simulink model "POWER_BTN_CONTROL"  (R2024b)
settings: configuration reference "MODEL_CONFIG_CHILD" (kept outside this file)
undefined symbols (not defined in the file): MILLI_SEC_COUNTS_10000_U16, MILLI_SEC_COUNTS_1000_U16, MILLI_SEC_COUNTS_2000_U16, SAMPLE_TIME_1MS
libraries: simulink x2
settings Model: DataDictionary=MCU_FOC_MAIN_DD.sldd  EnableAccessToBaseWorkspace=off  Creator=415  LastModifiedBy=415
settings ConfigSetRef: SourceName=MODEL_CONFIG_CHILD

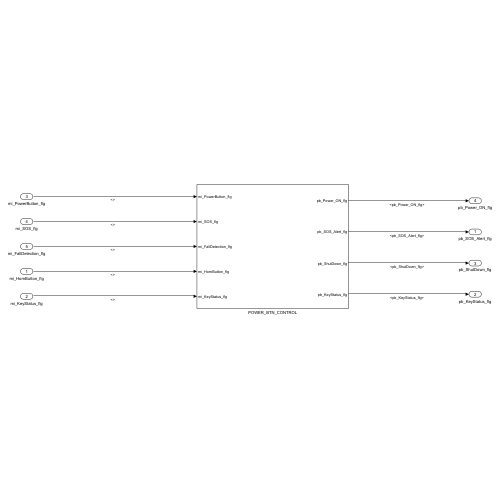
[thumbnail: Simulink's stored preview of the top-level diagram]
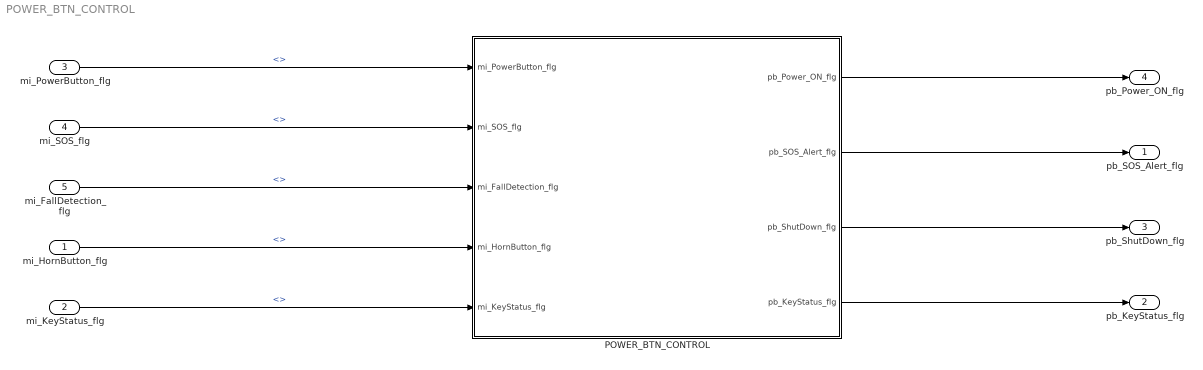
== system POWER_BTN_CONTROL ==
  mi_HornButton_flg : Inport
  mi_KeyStatus_flg : Inport  Port=2
  mi_PowerButton_flg : Inport  Port=3
  mi_SOS_flg : Inport  Port=4
  mi_FallDetection_flg : Inport  Port=5
  POWER_BTN_CONTROL : Subsystem
  pb_SOS_Alert_flg : Outport
  pb_KeyStatus_flg : Outport  Port=2
  pb_ShutDown_flg : Outport  Port=3
  pb_Power_ON_flg : Outport  Port=4
  wires:
  mi_PowerButton_flg/1 -> POWER_BTN_CONTROL/1(mi_PowerButton_flg)  "<>"
  POWER_BTN_CONTROL/3(pb_ShutDown_flg) -> pb_ShutDown_flg/1
  POWER_BTN_CONTROL/4(pb_KeyStatus_flg) -> pb_KeyStatus_flg/1
  POWER_BTN_CONTROL/1(pb_Power_ON_flg) -> pb_Power_ON_flg/1
  mi_KeyStatus_flg/1 -> POWER_BTN_CONTROL/5(mi_KeyStatus_flg)  "<>"
  POWER_BTN_CONTROL/2(pb_SOS_Alert_flg) -> pb_SOS_Alert_flg/1
  mi_FallDetection_flg/1 -> POWER_BTN_CONTROL/3(mi_FallDetection_flg)  "<>"
  mi_HornButton_flg/1 -> POWER_BTN_CONTROL/4(mi_HornButton_flg)  "<>"
  mi_SOS_flg/1 -> POWER_BTN_CONTROL/2(mi_SOS_flg)  "<>"

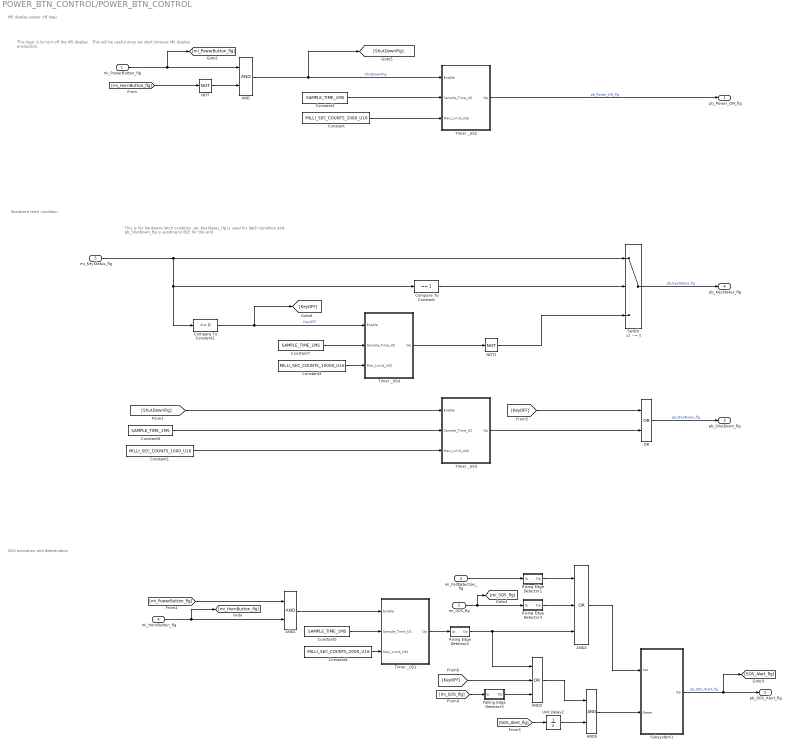
== system POWER_BTN_CONTROL/POWER_BTN_CONTROL ==
  note: This logic is to turn off the M5 display . This will be useful once we start inhouse M5 display production.
  note: M5 display power off logic
  note: This is for hardware latch condition .pb_KeyStatus_flg is used for latch condition and pb_ShutDown_flg is sending to BLE for trip end .
  note: Hardware latch condition
  note: SOS activation and deactivation
  mi_PowerButton_flg : Inport
  mi_SOS_flg : Inport  Port=2
  mi_FallDetection_flg : Inport  Port=3
  mi_HornButton_flg : Inport  Port=4
  mi_KeyStatus_flg : Inport  Port=5
  AND : Logic  AllPortsSameDT=off  OutDataTypeStr=boolean
  AND1 : Logic  AllPortsSameDT=off  OutDataTypeStr=boolean
  AND2 : Logic  Operator=OR  Inputs=3  AllPortsSameDT=off  OutDataTypeStr=boolean
  AND3 : Logic  Operator=OR  Inputs=3  AllPortsSameDT=off  OutDataTypeStr=boolean
  AND5 : Logic  AllPortsSameDT=off  OutDataTypeStr=boolean
  Compare To Constant : simulink/Logic and Bit Operations/Compare To Constant  relop===  const=1  OutDataTypeStr=boolean
  Compare To Constant1 : simulink/Logic and Bit Operations/Compare To Constant  relop===  const=0  OutDataTypeStr=boolean
  Constant : Constant  Value=MILLI_SEC_COUNTS_2000_U16
  Constant1 : Constant  Value=MILLI_SEC_COUNTS_1000_U16
  Constant{2,5,7..8} (4 alike) : Constant  Value=SAMPLE_TIME_1MS
  Constant3 : Constant  Value=MILLI_SEC_COUNTS_10000_U16
  Constant4 : Constant  Value=MILLI_SEC_COUNTS_2000_U16
  Falling Edge Detector3 : Subsystem
  NOT : Logic  Operator=NOT  AllPortsSameDT=off  OutDataTypeStr=boolean
  NOT1 : Logic  Operator=NOT  IconShape=distinctive  AllPortsSameDT=off  OutDataTypeStr=boolean
  OR : Logic  Operator=OR  AllPortsSameDT=off  OutDataTypeStr=boolean
  Rising Edge Detector1 : Subsystem
  Rising Edge Detector2 : Subsystem
  Rising Edge Detector3 : Subsystem
  Subsystem1 : Subsystem
  Switch : Switch  Criteria=u2 ~= 0  SaturateOnIntegerOverflow=off  InputSameDT=off
  Timer _US1 : Subsystem
  Timer _US2 : Subsystem
  Timer _US3 : Subsystem
  Timer _US4 : Subsystem
  Unit Delay2 : UnitDelay  SampleTime=-1  HasFrameUpgradeWarning=on
  pb_Power_ON_flg : Outport
  pb_SOS_Alert_flg : Outport  Port=2
  pb_ShutDown_flg : Outport  Port=3
  pb_KeyStatus_flg : Outport  Port=4
  wires:
  [KeyOFF] -> AND3/2
  OR/1 -> pb_ShutDown_flg/1  "pb_ShutDown_flg"
  [ShutDownFlg] -> Timer _US3/1(Enable)
  [KeyOFF] -> OR/1
  Compare To Constant/1 -> Switch/2
  Timer _US4/1(Op) -> NOT1/1
  NOT1/1 -> Switch/3
  Compare To Constant1/1 -> Timer _US4/1(Enable), [KeyOFF]  "KeyOFF"
  Switch/1 -> pb_KeyStatus_flg/1  "pb_KeyStatus_flg"
  mi_KeyStatus_flg/1 -> Compare To Constant/1, Compare To Constant1/1, Switch/1
  Constant7/1 -> Timer _US4/2(Sample_Time_US)
  Constant3/1 -> Timer _US4/3(Max_Limit_U32)
  Rising Edge Detector1/1(Op) -> AND2/1
  mi_FallDetection_flg/1 -> Rising Edge Detector1/1(Ip)
  Timer _US3/1(Op) -> OR/2
  Constant1/1 -> Timer _US3/3(Max_Limit_U32)
  Constant8/1 -> Timer _US3/2(Sample_Time_US)
  Unit Delay2/1 -> AND5/2
  [SOS_Alert_flg] -> Unit Delay2/1
  Rising Edge Detector3/1(Op) -> AND2/2
  [mi_SOS_flg] -> Falling Edge Detector3/1(Ip)
  AND5/1 -> Subsystem1/2(Reset)
  mi_SOS_flg/1 -> Rising Edge Detector3/1(Ip), [mi_SOS_flg]
  AND2/1 -> Subsystem1/1(Set)
  Rising Edge Detector2/1(Op) -> AND2/3, AND3/1
  AND1/1 -> Timer _US1/1(Enable)
  Constant5/1 -> Timer _US1/2(Sample_Time_US)
  Constant4/1 -> Timer _US1/3(Max_Limit_U32)
  Constant/1 -> Timer _US2/3(Max_Limit_U32)
  Constant2/1 -> Timer _US2/2(Sample_Time_US)
  AND/1 -> Timer _US2/1(Enable), [ShutDownFlg]  "ShutDownFlg"
  AND3/1 -> AND5/1
  Falling Edge Detector3/1(Op) -> AND3/3
  Subsystem1/1(Op) -> [SOS_Alert_flg], pb_SOS_Alert_flg/1  "pb_SOS_Alert_flg"
  Timer _US1/1(Op) -> Rising Edge Detector2/1(Ip)
  [mi_PowerButton_flg] -> AND1/1
  Timer _US2/1(Op) -> pb_Power_ON_flg/1  "pb_Power_ON_flg"
  NOT/1 -> AND/2
  [mi_HornButton_flg] -> NOT/1
  mi_HornButton_flg/1 -> [mi_HornButton_flg], AND1/2
  mi_PowerButton_flg/1 -> [mi_PowerButton_flg], AND/1

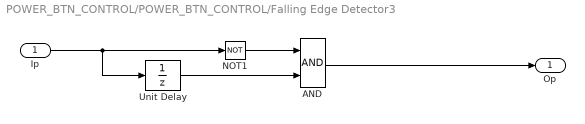
== system POWER_BTN_CONTROL/POWER_BTN_CONTROL/Falling Edge Detector3 ==
  Ip : Inport
  AND : Logic  AllPortsSameDT=off  OutDataTypeStr=boolean
  NOT1 : Logic  Operator=NOT  IconShape=distinctive  AllPortsSameDT=off  OutDataTypeStr=boolean
  Unit Delay : UnitDelay  SampleTime=-1  HasFrameUpgradeWarning=on
  Op : Outport
  wires:
  NOT1/1 -> AND/1
  Unit Delay/1 -> AND/2
  AND/1 -> Op/1
  Ip/1 -> NOT1/1, Unit Delay/1

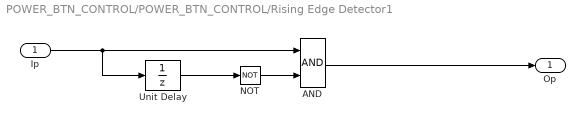
== system POWER_BTN_CONTROL/POWER_BTN_CONTROL/Rising Edge Detector1 ==
  Ip : Inport
  AND : Logic  AllPortsSameDT=off  OutDataTypeStr=boolean
  NOT : Logic  Operator=NOT  IconShape=distinctive  AllPortsSameDT=off  OutDataTypeStr=boolean
  Unit Delay : UnitDelay  SampleTime=-1  HasFrameUpgradeWarning=on
  Op : Outport
  wires:
  Ip/1 -> Unit Delay/1, AND/1
  AND/1 -> Op/1
  NOT/1 -> AND/2
  Unit Delay/1 -> NOT/1

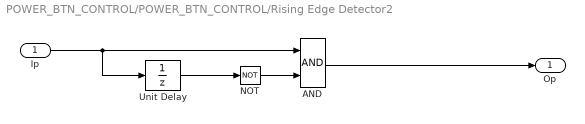
== system POWER_BTN_CONTROL/POWER_BTN_CONTROL/Rising Edge Detector2 ==
  Ip : Inport
  AND : Logic  AllPortsSameDT=off  OutDataTypeStr=boolean
  NOT : Logic  Operator=NOT  IconShape=distinctive  AllPortsSameDT=off  OutDataTypeStr=boolean
  Unit Delay : UnitDelay  SampleTime=-1  HasFrameUpgradeWarning=on
  Op : Outport
  wires:
  Ip/1 -> Unit Delay/1, AND/1
  AND/1 -> Op/1
  NOT/1 -> AND/2
  Unit Delay/1 -> NOT/1

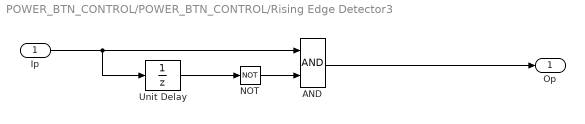
== system POWER_BTN_CONTROL/POWER_BTN_CONTROL/Rising Edge Detector3 ==
  Ip : Inport
  AND : Logic  AllPortsSameDT=off  OutDataTypeStr=boolean
  NOT : Logic  Operator=NOT  IconShape=distinctive  AllPortsSameDT=off  OutDataTypeStr=boolean
  Unit Delay : UnitDelay  SampleTime=-1  HasFrameUpgradeWarning=on
  Op : Outport
  wires:
  Unit Delay/1 -> NOT/1
  NOT/1 -> AND/2
  AND/1 -> Op/1
  Ip/1 -> AND/1, Unit Delay/1

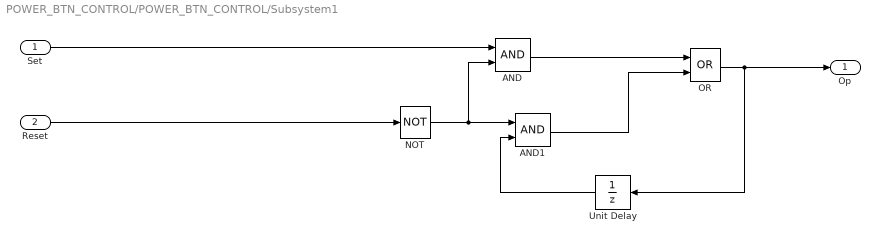
== system POWER_BTN_CONTROL/POWER_BTN_CONTROL/Subsystem1 ==
  Set : Inport
  Reset : Inport  Port=2
  AND : Logic  AllPortsSameDT=off  OutDataTypeStr=boolean
  AND1 : Logic  AllPortsSameDT=off  OutDataTypeStr=boolean
  NOT : Logic  Operator=NOT  IconShape=distinctive  AllPortsSameDT=off  OutDataTypeStr=boolean
  OR : Logic  Operator=OR  AllPortsSameDT=off  OutDataTypeStr=boolean
  Unit Delay : UnitDelay  SampleTime=-1  HasFrameUpgradeWarning=on
  Op : Outport
  wires:
  AND1/1 -> OR/2
  AND/1 -> OR/1
  Set/1 -> AND/1
  Unit Delay/1 -> AND1/2
  NOT/1 -> AND/2, AND1/1
  OR/1 -> Op/1, Unit Delay/1
  Reset/1 -> NOT/1

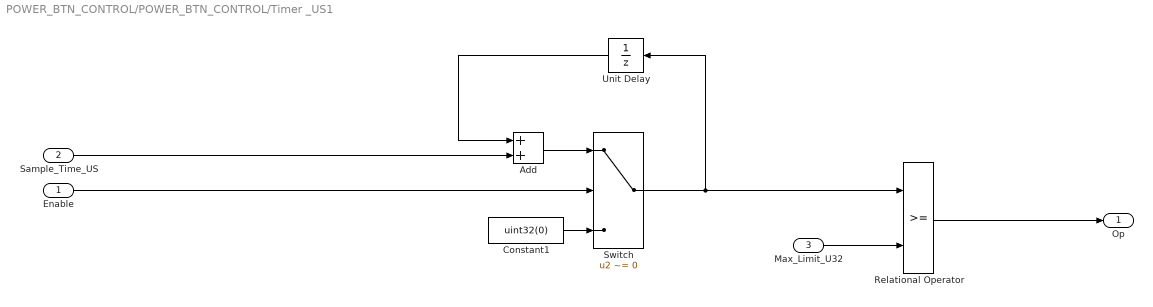
== system POWER_BTN_CONTROL/POWER_BTN_CONTROL/Timer _US1 ==
  Enable : Inport
  Sample_Time_US : Inport  Port=2
  Max_Limit_U32 : Inport  Port=3
  Add : Sum
  Constant1 : Constant  Value=uint32(0)
  Relational Operator : RelationalOperator  OutDataTypeStr=boolean  RndMeth=Simplest  InputSameDT=off
  Switch : Switch  Criteria=u2 ~= 0  SaturateOnIntegerOverflow=off  InputSameDT=off
  Unit Delay : UnitDelay  SampleTime=-1  HasFrameUpgradeWarning=on
  Op : Outport
  wires:
  Max_Limit_U32/1 -> Relational Operator/2
  Relational Operator/1 -> Op/1
  Enable/1 -> Switch/2
  Constant1/1 -> Switch/3
  Add/1 -> Switch/1
  Sample_Time_US/1 -> Add/2
  Unit Delay/1 -> Add/1
  Switch/1 -> Relational Operator/1, Unit Delay/1

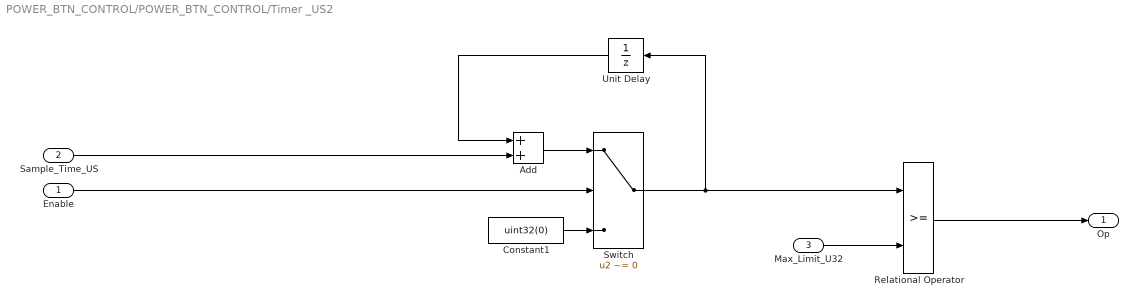
== system POWER_BTN_CONTROL/POWER_BTN_CONTROL/Timer _US2 ==
  Enable : Inport
  Sample_Time_US : Inport  Port=2
  Max_Limit_U32 : Inport  Port=3
  Add : Sum
  Constant1 : Constant  Value=uint32(0)
  Relational Operator : RelationalOperator  OutDataTypeStr=boolean  RndMeth=Simplest  InputSameDT=off
  Switch : Switch  Criteria=u2 ~= 0  SaturateOnIntegerOverflow=off  InputSameDT=off
  Unit Delay : UnitDelay  SampleTime=-1  HasFrameUpgradeWarning=on
  Op : Outport
  wires:
  Switch/1 -> Unit Delay/1, Relational Operator/1
  Unit Delay/1 -> Add/1
  Sample_Time_US/1 -> Add/2
  Add/1 -> Switch/1
  Constant1/1 -> Switch/3
  Enable/1 -> Switch/2
  Relational Operator/1 -> Op/1
  Max_Limit_U32/1 -> Relational Operator/2

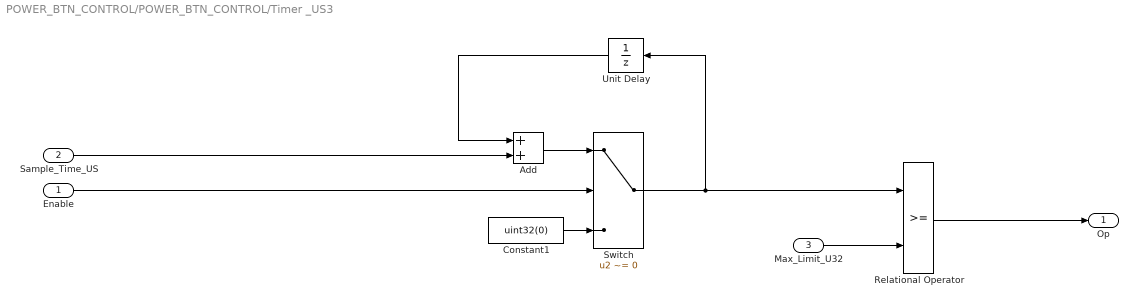
== system POWER_BTN_CONTROL/POWER_BTN_CONTROL/Timer _US3 ==
  Enable : Inport
  Sample_Time_US : Inport  Port=2
  Max_Limit_U32 : Inport  Port=3
  Add : Sum
  Constant1 : Constant  Value=uint32(0)
  Relational Operator : RelationalOperator  OutDataTypeStr=boolean  RndMeth=Simplest  InputSameDT=off
  Switch : Switch  Criteria=u2 ~= 0  SaturateOnIntegerOverflow=off  InputSameDT=off
  Unit Delay : UnitDelay  SampleTime=-1  HasFrameUpgradeWarning=on
  Op : Outport
  wires:
  Max_Limit_U32/1 -> Relational Operator/2
  Relational Operator/1 -> Op/1
  Enable/1 -> Switch/2
  Constant1/1 -> Switch/3
  Add/1 -> Switch/1
  Sample_Time_US/1 -> Add/2
  Unit Delay/1 -> Add/1
  Switch/1 -> Relational Operator/1, Unit Delay/1

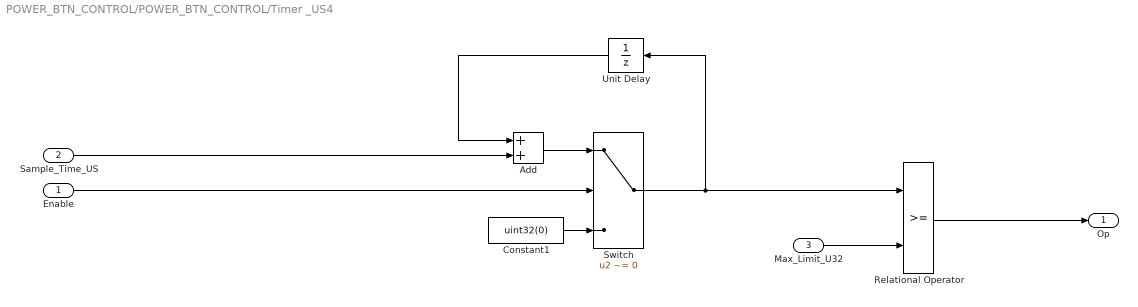
== system POWER_BTN_CONTROL/POWER_BTN_CONTROL/Timer _US4 ==
  Enable : Inport
  Sample_Time_US : Inport  Port=2
  Max_Limit_U32 : Inport  Port=3
  Add : Sum
  Constant1 : Constant  Value=uint32(0)
  Relational Operator : RelationalOperator  OutDataTypeStr=boolean  RndMeth=Simplest  InputSameDT=off
  Switch : Switch  Criteria=u2 ~= 0  SaturateOnIntegerOverflow=off  InputSameDT=off
  Unit Delay : UnitDelay  SampleTime=-1  HasFrameUpgradeWarning=on
  Op : Outport
  wires:
  Switch/1 -> Unit Delay/1, Relational Operator/1
  Unit Delay/1 -> Add/1
  Sample_Time_US/1 -> Add/2
  Add/1 -> Switch/1
  Constant1/1 -> Switch/3
  Enable/1 -> Switch/2
  Relational Operator/1 -> Op/1
  Max_Limit_U32/1 -> Relational Operator/2
